simulink model "joystick_and_autonomous_control"  (Simulink 8.2)
settings: Solver=FixedStepDiscrete  StartTime=0.0  StopTime=inf  FixedStep=0.04  RelTol=1e-3
libraries: etargetslib x17, simulink x13, dspnetwork x11, dspmtrx3 x10, xpcseriallib x7, visionsinks x2, visionstatistics x1, visiontextngfix x1, aerolibanimutils x1, SimulinkExecutionControl x1, instrumentlib x1
(part 2 of 2)

== system joystick_and_autonomous_control/Navigation Sensor Feedback/HoldSignal3/Enabled Subsystem ==
  In1 : Inport
  Enable : EnablePort
  Out1 : Outport
  wires:
  In1/1 -> Out1/1

== system joystick_and_autonomous_control/Navigation Sensor Feedback/HoldSignal4/Enabled Subsystem ==
  In1 : Inport
  Enable : EnablePort
  Out1 : Outport
  wires:
  In1/1 -> Out1/1

== system joystick_and_autonomous_control/Navigation Sensor Feedback/HoldSignal5/Enabled Subsystem ==
  In1 : Inport
  Enable : EnablePort
  Out1 : Outport
  wires:
  In1/1 -> Out1/1

== system joystick_and_autonomous_control/Navigation Sensor Feedback/HoldSignal6/Enabled Subsystem ==
  In1 : Inport
  Enable : EnablePort
  Out1 : Outport
  wires:
  In1/1 -> Out1/1

== matlab function Ball Tracking/MATLAB Function1 ==
  data: f1 input double; bwRed output double
function bwRed = redTracker(f1)
%#codegen

greyThreshold = 30;
rgThreshold = 20;
gbThreshold = 20;
rbThreshold = 20;

vidHeight = 144;
vidWidth = 176;

%RG channel
frg = f1(:, :, 1 : 2);
%GB channel
fgb = f1(:, :, 2 : 3);
%RB channel
frb = zeros(vidHeight, vidWidth, 2);
frb(:, :, 1) = f1(:, :, 1);
frb(:, :, 2) = f1(:, :, 3);

%null indexes
greynull = max(f1, [], 3) - min(f1, [], 3) < greyThreshold;
rgnull = max(frg, [], 3) - min(frg, [], 3) < rgThreshold;
gbnull = max(fgb, [], 3) - min(fgb, [], 3) < gbThreshold;
rbnull = max(frb, [], 3) - min(frb, [], 3) < rbThreshold;

%dominant indexes (GB null)
rdom = (max(f1, [], 3) - f1(:, :, 1)) < 1;


% f1_f = zeros(vidHeight, vidWidth, 2);
%red----------------------------
% fcred = f1(:, :, 1);
fcred = zeros(vidHeight, vidWidth);
fcred(rdom) = 255;

%strip greyscale
fcred(greynull) = 0;

%strip RG
fcred(rgnull) = 0;

%strip GB
fcred(gbnull & ~rdom) = 0;

%strip RB
fcred(rbnull) = 0;

%filter for R dominance
fcred(~rdom) = 0;

%reconstruct image
% f1_f(:, :, 1) = fcred;
bwRed = fcred;

== matlab function Landing Toggle/MATLAB Function ==
  data: toggle output double; u input double; add_last input double; adder output double; exit_u output double; u_last input double
function [toggle,adder,exit_u] = fcn(u,add_last,u_last)
%#codegen

% if u ~= last_u
% y = 1;
% else
% y = 0;    
% end
% 

if (u==64 & (u_last == 0))
    
   adder = add_last + 1;
%     exit_u = u;
else
    adder = add_last;
%     exit_u = u;
end

 exit_u = u;
 
 toggle=mod(adder,2);

% y = u;

== matlab function Joystick Controller/MATLAB Function ==
  data: u input double; roll output double; pitch output double
function [roll,pitch] = fcn(u)
%#codegen

if u == 0
    roll  = 0;
    pitch = -0.2;
%     yaw   = 
elseif u == 180
    roll  = 0;
    pitch = 0.2;
%     yaw   = 
    
elseif u == 90
    roll  = 0.2;
    pitch = 0;
%     yaw   = 
    
elseif u == 270
    roll  = -0.2;
    pitch = 0;
%     yaw   = 
else
    
    roll  = 0;
    pitch = 0;
%     yaw   = 0;
    
end

== stateflow chart Telemetry and Control ==
  state ExecuteTrimCmd_State
    entry:ErrorFlag = 0;
    during: sendTrim(i)
  state ModeSelector
  state sendTrim(DataStamp) [function]
  state WakeUpNavVideo_State
    entry:ErrorFlag = 0;
    during: WakeUpNav(i)
  state WakeUpNav(DataStamp) [function]
  state StartNavDemo_State
    entry:ErrorFlag = 0;
    during: StartNavDemo(i)
  state StartNavDemo(DataStamp) [function]
  state SetVideoChannel_State
    entry:ErrorFlag = 0;
    during: SetVideo(i)
  state SetVideo(DataStamp) [function]
  state BeginHover_State
    entry:ErrorFlag = 0;
    during: startHover(i);
  state startHover(DataStamp) [function]
  state RunMotor6
    entry:ErrorFlag = 0;
    during: sendLand(i);
  state sendLand(In1) [function]
  state Control_State
    entry:ErrorFlag = 0;
    entry: [VideoPackets,VidPackLen,NavPackets,NavPackLen]= sendAttVz(i,Active1,Roll,Pitch,Altitude,Yaw,i);
  state [VideoPackets,VidPackLen,NavPackets,NavPackLen] = sendAttVz(DataStamp_1,Active,Roll,Pitch,Altitude,Yaw,DataStamp_2) [function]
  state WaitStatic
    entry:ErrorFlag = 0;
    entry: [VideoPackets,VidPackLen,NavPackets,NavPackLen]= sendAttVz(i,0,0,0,0,0,i);
  (default) -> (junction 75)
  (junction 75) -> ModeSelector : {i = 1}
  ExecuteTrimCmd_State -> ModeSelector [order 1] : [mode~=4]
  ModeSelector -> ExecuteTrimCmd_State : [mode == 4]
      | {i=i+1;}
  ExecuteTrimCmd_State -> WakeUpNavVideo_State [order 2] : after(3,sec)
      | {i=i+1;}
  WaitStatic -> ModeSelector [order 1] : [mode ~= 4]
      | {i = i + 1;}
  RunMotor6 -> ModeSelector : after(1,sec)
  WakeUpNavVideo_State -> StartNavDemo_State : after(1,sec)
      | {i = i +1;}
  StartNavDemo_State -> SetVideoChannel_State : after(0.1,sec)
      | {i=i+1;}
  SetVideoChannel_State -> (junction 76) [order 2] : [staticFlag == 0]
  SetVideoChannel_State -> WaitStatic [order 1] : [staticFlag == 1]
  WaitStatic -> WaitStatic [order 2] : after(0.04, sec)
      | {i = i + 2;}
  (junction 76) -> BeginHover_State : after(0.1,sec)
      | {i =i +1;}
  Control_State -> RunMotor6 [order 1] : [mode~=4]
      | {i=i+1;}
  BeginHover_State -> Control_State : after(1,sec)
      | {i=i+2;}
  Control_State -> Control_State [order 2] : after(0.04,sec)
      | {i = i+2;}
  data: DataStamp function_input double; DataStamp function_input double; DataStamp function_input double; DataStamp function_input double; DataStamp function_input double; In1 function_input double; DataStamp_1 function_input double; Active function_input double; Roll function_input double; Pitch function_input double; Altitude function_input double; Yaw function_input double; DataStamp_2 function_input double; VideoPackets function_output double; VidPackLen function_output uint16; NavPackets function_output double; NavPackLen function_output double; Roll input double; Pitch input double; Altitude input double; Yaw input double; mode input double; i local double; NavPackets output uint8 size=[500,1]; NavPackLen output double; VideoPackets output uint8 size=[40000,1]; VidPackLen output uint16; ErrorFlag output double; Active1 input double; staticFlag input boolean

== stateflow chart Controller /Roll Pitch Decoupler ==
  state Idle
    entry:
    pitchactive = 0;
    rollactive = 0;
  state controlRoll
    entry:
    rollactive = 1;
    pitchactive = 0;
  state controlPitch
    entry:
    pitchactive = 1;
    rollactive = 0;
  state controlStart
  state controlEnd
    entry:
    pitchactive = 0;
    rollactive = 0;
  (default) -> Idle
  controlStart -> Idle [order 1] : [sqrt(abserrx^2 + abserry^2) <= 10]
  Idle -> controlStart : [sqrt(abserrx^2 + abserry^2) > 10]
  controlStart -> controlPitch [order 3] : [abserrx <= abserry]
  controlPitch -> controlEnd : [abserry < 5]
  controlStart -> controlRoll [order 2] : [abserrx > abserry]
  controlEnd -> controlStart : after(2, sec)
  controlRoll -> controlEnd : [abserrx < 5]
  data: abserrx input double; abserry input double; rollactive output double; pitchactive output double

== stateflow chart Controller /Operation Modes ==
  state DebugHover
    during:
    [roll_cmd,pitch_cmd,yaw_cmd, alt_cmd] = hover(dx,dy,dtheta,dx_dot,dy_dot,dtheta_dot,dalt,dalt_dot)
  state [roll_cmd,pitch_cmd,yaw_cmd,alt_cmd] = hover(e_x,e_y,e_theta,e_x_dot,e_y_dot,e_theta_dot,e_alt,e_alt_dot) [function]
  state WaitForNXT
    during:
    [roll_cmd,pitch_cmd,yaw_cmd, alt_cmd] = waitTrack(dx,dy,dtheta,dx_dot,dy_dot,dtheta_dot,dalt,dalt_dot)
  state [roll_cmd,pitch_cmd,yaw_cmd,alt_cmd] = waitTrack(e_x,e_y,e_theta,e_x_dot,e_y_dot,e_theta_dot,e_alt,e_alt_dot) [function]
  state NormalTracking
    during:
    [roll_cmd,pitch_cmd,yaw_cmd, alt_cmd] = track(dx,dy,dtheta,dx_dot,dy_dot,dtheta_dot,dalt,dalt_dot)
  state [roll_cmd,pitch_cmd,yaw_cmd,alt_cmd] = track(e_x,e_y,e_theta,e_x_dot,e_y_dot,e_theta_dot,e_alt,e_alt_dot) [function]
  state EndHover
    during:
    done_flag =1
  state LossTrack
    during:
    [roll_cmd,pitch_cmd,yaw_cmd, alt_cmd] = track(dx,dy,dtheta,dx_dot,dy_dot,dtheta_dot,dalt,dalt_dot)
  state InitializeGains
    entry:
  state FailureHover
    during:
    [roll_cmd,pitch_cmd,yaw_cmd, alt_cmd] = hover(dx,dy,dtheta,dx_dot,dy_dot,dtheta_dot,dalt,dalt_dot)
  (default) -> InitializeGains
  InitializeGains -> DebugHover
  DebugHover -> WaitForNXT
  WaitForNXT -> NormalTracking : [nxt_flag ==1]
  NormalTracking -> EndHover [order 2] : [nxt_destination ==1]
  NormalTracking -> LossTrack [order 1] : [nxt_flag ==0]
  LossTrack -> NormalTracking [order 1] : [nxt_flag==1]
  FailureHover -> NormalTracking : [nxt_flag==1]
  LossTrack -> FailureHover [order 2] : after(1.5, sec)
  data: e_x function_input double; e_y function_input double; e_theta function_input double; roll_cmd function_output double; pitch_cmd function_output double; yaw_cmd function_output double; e_x_dot function_input double; e_y_dot function_input double; e_theta_dot function_input double; e_alt function_input double; e_alt_dot function_input double; alt_cmd function_output double; e_x function_input double; e_y function_input double; e_theta function_input double; roll_cmd function_output double; pitch_cmd function_output double; yaw_cmd function_output double; e_x_dot function_input double; e_y_dot function_input double; e_theta_dot function_input double; e_alt function_input double; e_alt_dot function_input double; alt_cmd function_output double; e_x function_input double; e_y function_input double; e_theta function_input double; roll_cmd function_output double; pitch_cmd function_output double; yaw_cmd function_output double; e_x_dot function_input double; e_y_dot function_input double; e_theta_dot function_input double; e_alt function_input double; e_alt_dot function_input double; alt_cmd function_output double; dx input double; dy input double; dtheta input double; pitch_cmd output double; yaw_cmd output double; roll_cmd output double; alt_cmd output double; dalt input double; done_flag output boolean; nxt_flag input boolean; nxt_destination input boolean; dx_dot input double; dy_dot input double; dtheta_dot input double; dalt_dot input double; K_wait local double; K_dot_wait local double =0; K_track local double =0; K_dot_track local double size=[1 4]; NormalTracking output boolean; LossTrack output boolean; FailureHover1 output boolean
